simulink model "PIDBLOCK"  (R2020b)
settings: Solver=FixedStepDiscrete  StartTime=0.0  StopTime=2  RelTol=1e-3
undefined symbols (not defined in the file): sigbuilder_block, tf5
libraries: pid_lib x1
settings Model: DataTypeOverride=Off  FPTShortcutValueString='{{},{''BaselineRun'',1,1,1,''BaselineRun'','''',{},''M'','''',''''},{''BaselineRun_2'',1,1,1,''BaselineRun_2'','''',{},''M'','''',''''}}'  Creator=EMRE  LastModifiedBy=EMRE
settings OptimizationCC: BlockReduction=off  ConditionallyExecuteInputs=off  DefaultParameterBehavior=Inlined
settings DebuggingCC: SignalRangeChecking=warning  AlgebraicLoopMsg=error  SingleTaskRateTransMsg=error
settings HardwareCC: ProdBitPerPointer=32  ProdBitPerSizeT=32  ProdBitPerPtrDiffT=32  ProdLargestAtomicFloat=None  ProdIntDivRoundTo=Undefined  ProdEndianess=Unspecified  ProdWordSize=32  ProdHWDeviceType=ASIC/FPGA->ASIC/FPGA  TargetBitPerPointer=64  TargetBitPerSizeT=64  TargetBitPerPtrDiffT=64  TargetLongLongMode=on  TargetIntDivRoundTo=Zero  TargetEndianess=LittleEndian  TargetWordSize=64  TargetHWDeviceType=Custom Processor->MATLAB Host Computer  ProdEqTarget=off

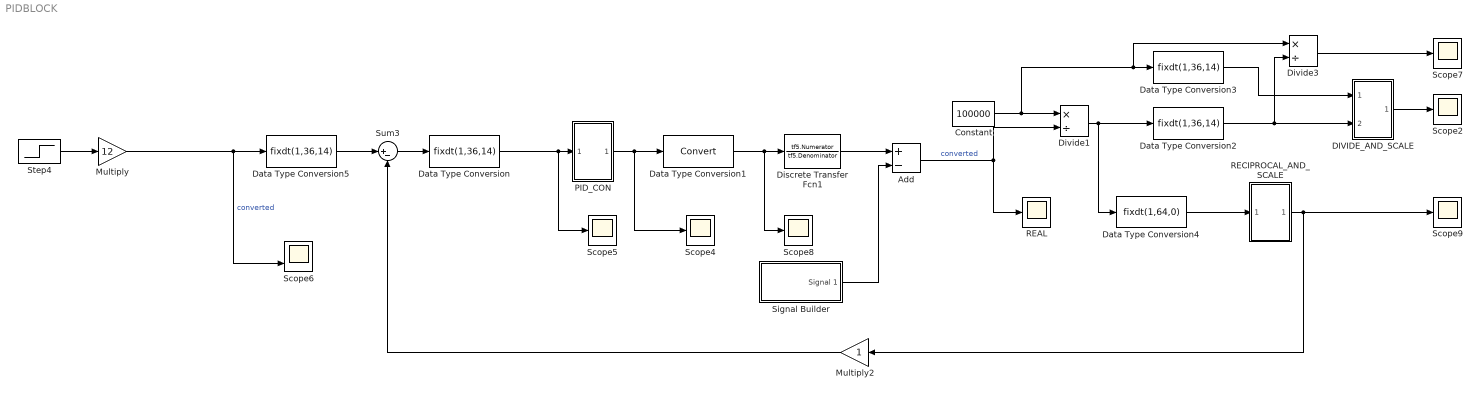
== system PIDBLOCK ==
  Add : Sum  Inputs=+-
  Constant : Constant  Value=100000
  DIVIDE_AND_SCALE : Subsystem
  Data Type Conversion{,2..3,5} (4 alike) : DataTypeConversion  OutDataTypeStr=fixdt(1,36,14)
  Data Type Conversion1 : DataTypeConversion
  Data Type Conversion4 : DataTypeConversion  OutDataTypeStr=fixdt(1,64,0)  SaturateOnIntegerOverflow=on
  Discrete Transfer Fcn1 : DiscreteTransferFcn  Numerator=tf5.Numerator  Denominator=tf5.Denominator  SampleTime=tf5.Ts
  Divide1 : Product  Inputs=*/  RndMeth=Zero  SaturateOnIntegerOverflow=on
  Divide3 : Product  Inputs=*/  OutMin=0  OutMax=25  RndMeth=Zero  SaturateOnIntegerOverflow=on
  Multiply : Gain  Gain=12
  Multiply2 : Gain
  PID_CON : Subsystem
  REAL : Scope
  RECIPROCAL_AND_SCALE : Subsystem
  Scope{2,4..5,7..9} (6 alike) : Scope
  Scope6 : Scope  NumInputPorts=2
  Signal Builder : Subsystem  Tag=STV Subsys  LoadFcn=sigbuilder_block('load');  StartFcn=sigbuilder_block('start');  StopFcn=sigbuilder_block('stop');  ClipboardFcn=sigbuilder_block('clipboard');  mask(Sigbuilder block){tuvar=[0:10]}
      mask help: Simulink:masks:SigbuilderBlock_MD
      mask init:
      | if ~strcmp(get_param(bdroot(gcbh),'SimulationStatus'),'stopped') tuvar = sigbuilder_block('maskInit'); end
      settings: CopyFcn=sigbuilder_block('copy');  DeleteFcn=sigbuilder_block('delete');  ModelCloseFcn=sigbuilder_block('modelClose');  PreSaveFcn=sigbuilder_block('preSave');  PauseFcn=sigbuilder_block('pause');  ContinueFcn=sigbuilder_block('continue');  NameChangeFcn=sigbuilder_block('namechange');  OpenFcn=sigbuilder_block('open',[437.6 199.2 550.4 400 ]);  CloseFcn=sigbuilder_block('close');
      mask Display: plot(0, 0, 100, 100,[2, 2, 32, 32, 2], [68, 8, 8, 68, 68],[32, 2], [38, 38], [32, 19, 2],[53, 60, 44], [32, 17, 17, 2],[16, 16, 31, 31]);txt = getActiveGroup(gcbh);text(2, 100, txt,'verticalAlignment', 'top');
  Step4 : Step  Time=0.2  SampleTime=0
  Sum3 : Sum  Inputs=|+-
  wires:
  Multiply/1 -> Data Type Conversion5/1, Scope6/2  "converted"
  Step4/1 -> Multiply/1
  Discrete Transfer Fcn1/1 -> Add/1
  Signal Builder/1(Signal 1) -> Add/2
  Add/1 -> REAL/1, Divide1/2  "converted"
  Sum3/1 -> Data Type Conversion/1
  PID_CON/1(PID_OUT) -> Data Type Conversion1/1, Scope4/1
  Data Type Conversion/1 -> PID_CON/1(PID_IN), Scope5/1
  Data Type Conversion1/1 -> Discrete Transfer Fcn1/1, Scope8/1
  Data Type Conversion2/1 -> DIVIDE_AND_SCALE/2(In2), Divide3/2
  Constant/1 -> Divide3/1, Data Type Conversion3/1, Divide1/1
  Divide3/1 -> Scope7/1
  DIVIDE_AND_SCALE/1(Out1) -> Scope2/1
  Data Type Conversion3/1 -> DIVIDE_AND_SCALE/1(In1)
  Multiply2/1 -> Sum3/2
  Divide1/1 -> Data Type Conversion4/1, Data Type Conversion2/1
  RECIPROCAL_AND_SCALE/1(Out1) -> Scope9/1, Multiply2/1
  Data Type Conversion4/1 -> RECIPROCAL_AND_SCALE/1(In1)
  Data Type Conversion5/1 -> Sum3/1

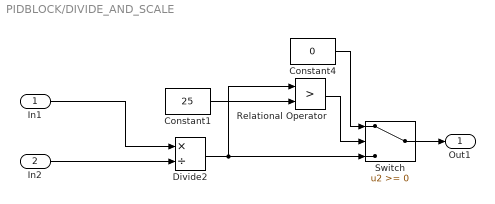
== system PIDBLOCK/DIVIDE_AND_SCALE ==
  In1 : Inport
  In2 : Inport  Port=2
  Constant1 : Constant  Value=25  OutDataTypeStr=fixdt(1,36,0)
  Constant4 : Constant  Value=0  OutDataTypeStr=fixdt(1,36,0)
  Divide2 : Product  Inputs=*/  OutMin=0  OutMax=25  OutDataTypeStr=fixdt(1,36,0)  RndMeth=Zero  SaturateOnIntegerOverflow=on
  Relational Operator : RelationalOperator  Operator=>  OutDataTypeStr=boolean  RndMeth=Simplest
  Switch : Switch  OutDataTypeStr=fixdt(1,36,0)
  Out1 : Outport
  wires:
  Switch/1 -> Out1/1
  Constant1/1 -> Relational Operator/2
  Constant4/1 -> Switch/1
  Relational Operator/1 -> Switch/2
  Divide2/1 -> Relational Operator/1, Switch/3
  In2/1 -> Divide2/2
  In1/1 -> Divide2/1

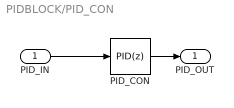
== system PIDBLOCK/PID_CON ==
  PID_IN : Inport
  PID_CON : pid_lib/PID Controller  Controller=PID  Form=Parallel  TimeDomain=Discrete-time  UseExternalTs=off  SampleTime=1/1430  IntegratorMethod=Forward Euler  FilterMethod=Forward Euler  ControllerParametersSource=internal  P=607.01219758038  I=32058.2249087534  D=-0.822082297791843  UseFilter=on  N=340.735232426423  TunerSelectOption=Transfer Function Based (PID Tuner App)  InitialConditionSource=internal  InitialConditionForIntegrator=1  InitialConditionForFilter=1  DifferentiatorICPrevScaledInput=0  ExternalReset=none  TrackingMode=off  Kt=1  LimitOutput=on  SatLimitsSource=internal  UpperSaturationLimit=10000  LowerSaturationLimit=0  LinearizeAsGain=off  AntiWindupMode=none  Kb=1  PGainOutDataTypeStr=fixdt(1,36,14)  PProdOutDataTypeStr=fixdt(1,36,14)  POutMin=[]  POutMax=[]  IGainOutDataTypeStr=fixdt(1,36,14)  IProdOutDataTypeStr=fixdt(1,36,14)  IOutMin=[]  IOutMax=[]  DGainOutDataTypeStr=fixdt(1,36,14)  DProdOutDataTypeStr=fixdt(1,36,14)  DOutMin=[]  DOutMax=[]  NGainOutDataTypeStr=fixdt(1,36,14)  NProdOutDataTypeStr=fixdt(1,36,14)  NOutMin=[]  NOutMax=[]  SumOutDataTypeStr=fixdt(1,36,14)  SumOutMin=[]  SumOutMax=[]  SaturationOutDataTypeStr=fixdt(1,36,14)  SaturationOutMin=[]  SaturationOutMax=[]  PParamMin=[]  PParamMax=[]  IParamMin=[]  IParamMax=[]  DParamMin=[]  DParamMax=[]  NParamMin=[]  NParamMax=[]  KbParamMin=[]  KbParamMax=[]  KtParamMin=[]  KtParamMax=[]  KbOutMin=[]  KbOutMax=[]  KtOutMin=[]  KtOutMax=[]  IntegratorOutDataTypeStr=fixdt(0,16,1)  IntegratorOutMin=[]  IntegratorOutMax=[]  FilterOutDataTypeStr=fixdt(1,16,12)  FilterOutMin=[]  FilterOutMax=[]  SumI1OutMin=[]  SumI1OutMax=[]  SumI2OutMin=[]  SumI2OutMax=[]  SumI3OutMin=[]  SumI3OutMax=[]  SumI4OutMin=[]  SumI4OutMax=[]  SumDOutDataTypeStr=fixdt(1,16,11)  SumDOutMin=[]  SumDOutMax=[]  DifferentiatorOutMin=[]  DifferentiatorOutMax=[]  FilterDiffOutCoefMin=[]  FilterDiffOutCoefMax=[]  ReciprocalOutMin=[]  ReciprocalOutMax=[]  SumDenOutMin=[]  SumDenOutMax=[]  SumNumOutMin=[]  SumNumOutMax=[]  DivideOutMin=[]  DivideOutMax=[]  UdiffTsProdOutMin=[]  UdiffTsProdOutMax=[]  NTsProdOutMin=[]  NTsProdOutMax=[]  UintegralTsProdOutMin=[]  UintegralTsProdOutMax=[]  UngainTsProdOutMin=[]  UngainTsProdOutMax=[]  IntegratorContinuousStateAttributes=''  IntegratorStateMustResolveToSignalObject=off  IntegratorRTWStateStorageClass=Auto  FilterContinuousStateAttributes=''  FilterStateMustResolveToSignalObject=off  FilterRTWStateStorageClass=Auto  ParallelPVariant=InternalParameters  IdealPVariant=Disabled  IVariant=InternalParameters  DVariant=InternalParameters  IntegratorVariant=Discrete  SatVariant=Enabled  AWVariant=Passthrough  PCopyVariant=Disabled  TRVariant=Disabled  FdbkBlocksVariant=Forward  IdealPFdbkVariant=Disabled  SatFdbkVariant=Disabled  DerivativeFilterVariant=ForwardEulerFilter  NVariant=InternalParameters  NCopyVariant=Disabled  FilterICVariant=InternalICsFilter  IntegratorICVariant=InternalICs  ExternalResetVariant=Disabled  TRSumVariant=Passthrough  SumFdbkVariant=Disabled  SumVariant=Sum_PID  TsampFilterVariant=InternalTs  TsampNgainVariant=Passthrough  TsampIntegralVariant=Passthrough  ExternalSaturationOutDataTypeStr=Inherit: Same as second input
  PID_OUT : Outport
  wires:
  PID_CON/1 -> PID_OUT/1
  PID_IN/1 -> PID_CON/1

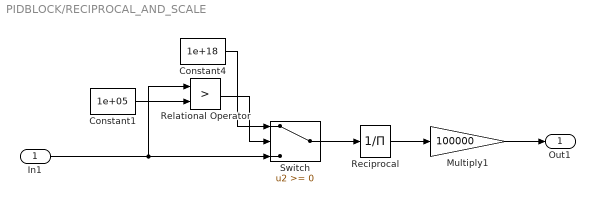
== system PIDBLOCK/RECIPROCAL_AND_SCALE ==
  In1 : Inport
  Constant1 : Constant  Value=1e+05  OutDataTypeStr=fixdt(1,64,0)
  Constant4 : Constant  Value=1e+18  OutDataTypeStr=fixdt(1,64,0)
  Multiply1 : Gain  Gain=100000  OutDataTypeStr=fixdt(1,36,14)
  Reciprocal : Product  Inputs=/  OutDataTypeStr=fixdt(1,36,30)  RndMeth=Zero  SaturateOnIntegerOverflow=on
  Relational Operator : RelationalOperator  Operator=>  OutDataTypeStr=boolean  RndMeth=Simplest
  Switch : Switch  OutDataTypeStr=fixdt(1,64,0)
  Out1 : Outport
  wires:
  In1/1 -> Switch/3, Relational Operator/1
  Relational Operator/1 -> Switch/2
  Reciprocal/1 -> Multiply1/1
  Switch/1 -> Reciprocal/1
  Constant4/1 -> Switch/1
  Constant1/1 -> Relational Operator/2
  Multiply1/1 -> Out1/1

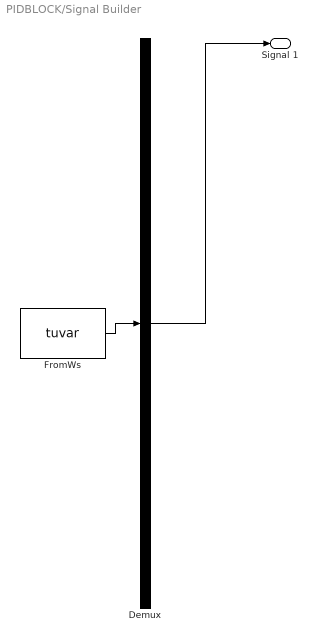
== system PIDBLOCK/Signal Builder ==
  Demux : Demux  Tag=STV Demux  Outputs=1
      settings: DisplayOption=none
  FromWs : FromWorkspace  Tag=STV FromWs  VariableName=tuvar
      SigBuilderData=|
      | common.afterFinalStr = 'Extrapolate'
      | common.sampleTime = 0
      | dataSet.timeRange = [0 2]
      | dataSet.name = 'Group 1'
      | sbobj.Groups.Name = 'Group 1'
      | sbobj.Groups.Signals.Name = 'Signal 1'
      | sbobj.Groups.Signals.XData = [0 0.7 0.7 0.7 0.7 0.75 0.75 0.8 0.8 2]
      | sbobj.Groups.Signals.YData = [0 0 0.24 0.905 0.425 0.425 0.9 0.9 0.01 0]
      | sbobj.Groups.TimeRange = [0 2]
  Signal 1 : Outport  Tag=STV Outport
  wires:
  Demux/1 -> Signal 1/1
  FromWs/1 -> Demux/1
